simulink model "mymemristortest"  (R2025a)
settings: Solver=VariableStepAuto  StartTime=0.0  StopTime=10.0  RelTol=1e-3
settings Model: PacingRate=0.001000  Creator=rr722  LastModifiedBy=rr722

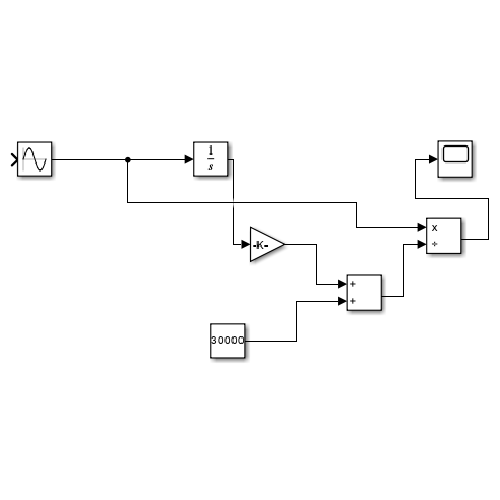
[thumbnail: Simulink's stored preview of the top-level diagram]
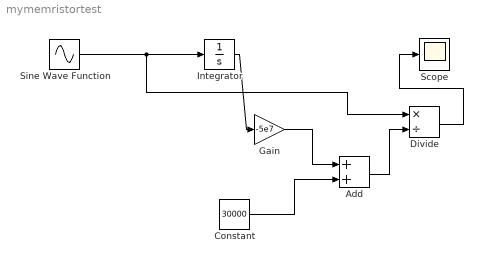
== system mymemristortest ==
  Add : Sum
  Constant : Constant  Value=30000
  Divide : Product  Inputs=*/
  Gain : Gain  Gain=-5e7
  Integrator : Integrator
  Scope : Scope
  Sine Wave Function : Sin  TimeSource=Use external signal  Amplitude=1.5  Frequency=2*pi*60  SampleTime=0
  wires:
  Integrator/1 -> Gain/1
  Gain/1 -> Add/1
  Constant/1 -> Add/2
  Add/1 -> Divide/2
  Sine Wave Function/1 -> Divide/1, Integrator/1
  Divide/1 -> Scope/1
